simulink model "SimulinkCFARHDLWorkflowExampleNew0710"  (R2022a)
settings: Solver=FixedStepDiscrete  StartTime=0.0  StopTime=T  RelTol=1e-3
PreLoadFcn:
  | rng default;
  | 
  | %% Parameters
  | Ncell = 1000;
  | NoTrainingCells = 50; % On One Side
  | NoGuardCells = 2; %On One Side
  | ProbabilityFalseAlarm = 0.005;
  | 
  | %% Stop Time
  | tstop = Ncell;
  | Latency = NoTrainingCells + NoGuardCells + NoTrainingCells + 16 + 7;
  | T = tstop + Latency;
  | 
  | 
  | %% Input
  | x = 1/sqrt(2)*(randn(1,Ncell) + 1i*randn(1,Ncell));
  | S = [x zeros(1,Latency)]; % Padding Zeros for Streaming
  | 
  | %% Fixed Point
  | 
  | FixedPointWord = 24;
  | FractionLength = 12;
  | Signed = 1;
undefined symbols (not defined in the file): y_t1
libraries: phaseddetectlib x1
settings Model: DataTypeOverride=Off  PauseTimes=1118  Creator=The MathWorks, Inc.  LastModifiedBy=vboxuser
settings SolverCC: AlgebraicLoopSolver=TrustRegion  MaxZcPerStep=1
settings OptimizationCC: BlockReduction=off  ConditionallyExecuteInputs=off  DefaultParameterBehavior=Inlined
settings DebuggingCC: AlgebraicLoopMsg=error  SingleTaskRateTransMsg=error  IntegerOverflowMsg=none  ParameterPrecisionLossMsg=none  UnconnectedInputMsg=warning  UnconnectedOutputMsg=warning  UnconnectedLineMsg=warning  SFMachineParentedDataDiag=warning
settings HardwareCC: ProdBitPerPointer=32  ProdBitPerSizeT=32  ProdBitPerPtrDiffT=32  ProdLargestAtomicFloat=None  ProdIntDivRoundTo=Undefined  ProdEndianess=Unspecified  ProdWordSize=32  ProdHWDeviceType=ASIC/FPGA->ASIC/FPGA  TargetBitPerPointer=64  TargetBitPerSizeT=64  TargetBitPerPtrDiffT=64  TargetLongLongMode=on  TargetIntDivRoundTo=Zero  TargetEndianess=LittleEndian  TargetWordSize=64  TargetHWDeviceType=Custom Processor->MATLAB Host Computer  ProdEqTarget=off
settings RTWCC: DLArmComputeVersion=19.05

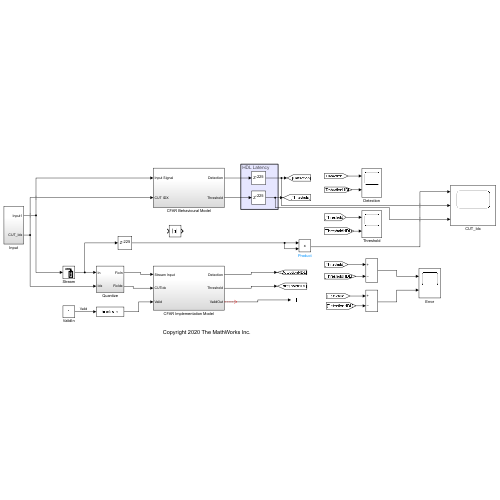
[thumbnail: Simulink's stored preview of the top-level diagram]
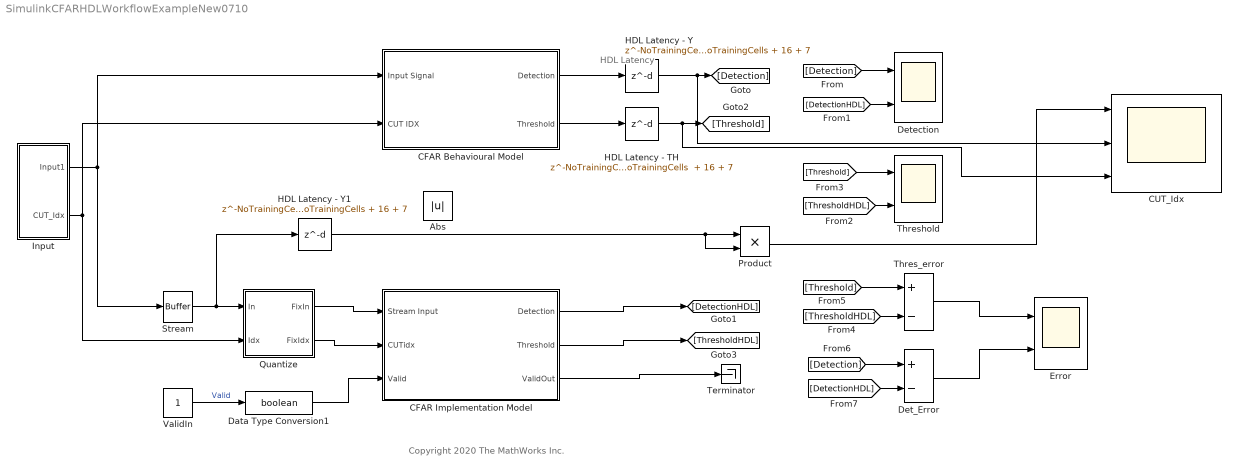
== system SimulinkCFARHDLWorkflowExampleNew0710 ==
  note: Copyright 2020 The MathWorks Inc.
  note: HDL Latency
  Abs : Abs  SaturateOnIntegerOverflow=off
  CFAR Behavioural Model : Subsystem
  CFAR Implementation Model : Subsystem
  "CUT_Idx " : Scope  NumInputPorts=3
  Data Type Conversion1 : DataTypeConversion  OutDataTypeStr=boolean  SaturateOnIntegerOverflow=off  RndMeth=Floor
  Det_Error : Sum  Inputs=+-
  Detection : Scope  NumInputPorts=2
  Error : Scope  NumInputPorts=2
  HDL Latency - TH : Delay  DelayLength="NoTrainingCells + NoGuardCells + NoTrainingCells  + 16 + 7"
  HDL Latency - Y : Delay  DelayLength=NoTrainingCells + NoGuardCells + NoTrainingCells + 16 + 7
  HDL Latency - Y1 : Delay  DelayLength=NoTrainingCells + NoGuardCells + NoTrainingCells + 16 + 7
  Input : Subsystem
  Product : Product
  Quantize : Subsystem
  Stream : Buffer  N=1  OutputFrames=off
  Terminator : Terminator
  Thres_error : Sum  Inputs=+-
  Threshold : Scope  NumInputPorts=2
  ValidIn : Constant  SampleTime=1
  wires:
  HDL Latency - Y/1 -> "CUT_Idx "/2, [Detection]
  HDL Latency - TH/1 -> "CUT_Idx "/3, [Threshold]
  Thres_error/1 -> Error/1
  Det_Error/1 -> Error/2
  [Detection] -> Detection/1
  [DetectionHDL] -> Detection/2
  [ThresholdHDL] -> Threshold/2
  [Threshold] -> Threshold/1
  [ThresholdHDL] -> Thres_error/2
  [Threshold] -> Thres_error/1
  [Detection] -> Det_Error/1
  [DetectionHDL] -> Det_Error/2
  Stream/1 -> HDL Latency - Y1/1, Quantize/1(In)
  CFAR Implementation Model/2(Threshold) -> [ThresholdHDL]
  CFAR Implementation Model/1(Detection) -> [DetectionHDL]
  Quantize/1(FixIn) -> CFAR Implementation Model/1(Stream Input)
  Quantize/2(FixIdx) -> CFAR Implementation Model/2(CUTidx)
  ValidIn/1 -> Data Type Conversion1/1  "Valid"
  CFAR Implementation Model/3(ValidOut) -> Terminator/1
  Data Type Conversion1/1 -> CFAR Implementation Model/3(Valid)
  CFAR Behavioural Model/1(Detection) -> HDL Latency - Y/1
  CFAR Behavioural Model/2(Threshold) -> HDL Latency - TH/1
  Input/1(Input1) -> CFAR Behavioural Model/1(Input Signal), Stream/1
  Input/2(CUT_Idx) -> CFAR Behavioural Model/2(CUT IDX), Quantize/2(Idx)
  Product/1 -> "CUT_Idx "/1
  HDL Latency - Y1/1 -> Product/2, Product/1
  ? -> ?

== system SimulinkCFARHDLWorkflowExampleNew0710/CFAR Behavioural Model ==
  Input Signal : Inport
  CUT IDX : Inport  Port=2
  CFAR Detector : phaseddetectlib/CFAR Detector  Method=CA  Rank=1  NumGuardCells=NoGuardCells*2  NumTrainingCells=NoTrainingCells*2  ThresholdFactor=Auto  ProbabilityFalseAlarm=ProbabilityFalseAlarm  CustomThresholdFactor=1  OutputFormat=CUT result  ThresholdOutputPort=on  NoisePowerOutputPort=off  NumDetectionsSource=Auto  NumDetections=1  SimulateUsing=Interpreted execution
      settings: SourceProductBaseCode=AR
  Selector1 : Selector  InputPortWidth=T  IndexOptions=Index vector (dialog)  Indices=1:Ncell  OutputSizes=1
  SquareLaw : Subsystem
  Detection : Outport
  Threshold : Outport  Port=2
  wires:
  CFAR Detector/1 -> Detection/1
  CFAR Detector/2 -> Threshold/1
  SquareLaw/1(SQR_LAW) -> CFAR Detector/1
  CUT IDX/1 -> CFAR Detector/2
  Input Signal/1 -> Selector1/1
  Selector1/1 -> SquareLaw/1(input)

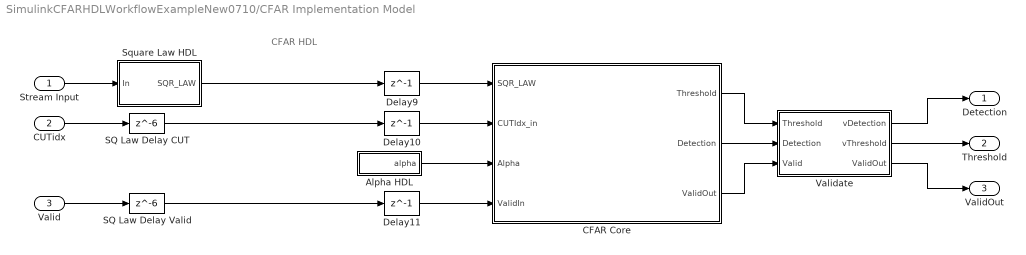
== system SimulinkCFARHDLWorkflowExampleNew0710/CFAR Implementation Model ==
  note: CFAR HDL
  Stream Input : Inport
  CUTidx : Inport  Port=2
  Valid : Inport  Port=3
  Alpha HDL : Subsystem
  CFAR Core : Subsystem
  Delay10 : Delay  DelayLength=1
  Delay11 : Delay  DelayLength=1
  Delay9 : Delay  DelayLength=1
  SQ Law Delay CUT : Delay  DelayLength=6
  SQ Law Delay Valid : Delay  DelayLength=6
  Square Law HDL : Subsystem
  Validate : Subsystem
  Detection : Outport
  Threshold : Outport  Port=2
  ValidOut : Outport  Port=3
  wires:
  Stream Input/1 -> Square Law HDL/1(In)
  Validate/3(ValidOut) -> ValidOut/1
  Validate/1(vDetection) -> Detection/1
  CUTidx/1 -> SQ Law Delay CUT/1
  Validate/2(vThreshold) -> Threshold/1
  Valid/1 -> SQ Law Delay Valid/1
  CFAR Core/3(ValidOut) -> Validate/3(Valid)
  Square Law HDL/1(SQR_LAW) -> Delay9/1
  SQ Law Delay CUT/1 -> Delay10/1
  CFAR Core/1(Threshold) -> Validate/1(Threshold)
  Alpha HDL/1(alpha) -> CFAR Core/3(Alpha)
  Delay11/1 -> CFAR Core/4(ValidIn)
  CFAR Core/2(Detection) -> Validate/2(Detection)
  Delay10/1 -> CFAR Core/2(CUTIdx_in)
  SQ Law Delay Valid/1 -> Delay11/1
  Delay9/1 -> CFAR Core/1(SQR_LAW)

== system SimulinkCFARHDLWorkflowExampleNew0710/Input ==
  CUT : Subsystem
  Input : Constant  Value=S
  Input2 : Constant  Value=y_t1
  Input1 : Outport
  CUT_Idx : Outport  Port=2
  wires:
  CUT/1(CUT_ref) -> CUT_Idx/1  "CUT_Idx"
  Input2/1 -> Input1/1  "Input"

== system SimulinkCFARHDLWorkflowExampleNew0710/Quantize ==
  In : Inport
  Idx : Inport  Port=2
  Fixed_Point_Idx : DataTypeConversion  OutDataTypeStr=fixdt(1,16,0)  SaturateOnIntegerOverflow=off  RndMeth=Floor
  Fixed_Point_Input : DataTypeConversion  OutDataTypeStr=fixdt(1,FixedPointWord,FractionLength)  SaturateOnIntegerOverflow=off  RndMeth=Floor
  FixIn : Outport
  FixIdx : Outport  Port=2
  wires:
  Fixed_Point_Input/1 -> FixIn/1
  Fixed_Point_Idx/1 -> FixIdx/1
  In/1 -> Fixed_Point_Input/1
  Idx/1 -> Fixed_Point_Idx/1

== system SimulinkCFARHDLWorkflowExampleNew0710/CFAR Behavioural Model/SquareLaw ==
  input : Inport
  Complex to Real-Imag : ComplexToRealImag
  a.a : Product
  a.a + b.b : Sum
  b.b : Product
  SQR_LAW : Outport
  wires:
  input/1 -> Complex to Real-Imag/1
  Complex to Real-Imag/2 -> b.b/1, b.b/2
  a.a/1 -> a.a + b.b/1
  a.a + b.b/1 -> SQR_LAW/1  "SQR_LAW"
  b.b/1 -> a.a + b.b/2
  Complex to Real-Imag/1 -> a.a/2, a.a/1

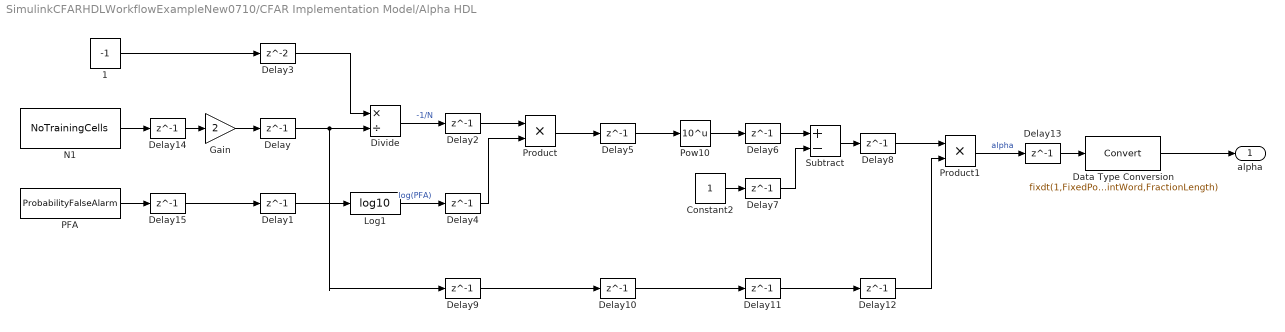
== system SimulinkCFARHDLWorkflowExampleNew0710/CFAR Implementation Model/Alpha HDL ==
  1 : Constant  Value=-1  OutDataTypeStr=Inherit: Inherit via back propagation  SampleTime=1
  Constant2 : Constant  OutDataTypeStr=Inherit: Inherit via back propagation  SampleTime=1
  Data Type Conversion : DataTypeConversion  OutDataTypeStr=fixdt(1,FixedPointWord,FractionLength)  SaturateOnIntegerOverflow=off  RndMeth=Floor
  Delay{,1..2,4..15} (15 alike) : Delay  DelayLength=1  InitialCondition=1
  Delay3 : Delay  InitialCondition=1
  Divide : Product  Inputs=*/  InputSameDT=on  RndMeth=Simplest  SaturateOnIntegerOverflow=on
  Gain : Gain  Gain=2
  Log1 : Math  Operator=log10  SignedPower=on  RndMeth=Zero
  N1 : Constant  Value=NoTrainingCells  OutDataTypeStr=single  SampleTime=1
  PFA : Constant  Value=ProbabilityFalseAlarm  OutDataTypeStr=single  SampleTime=1
  Pow10 : Math  Operator=10^u  SignedPower=on  RndMeth=Zero
  Product : Product
  Product1 : Product
  Subtract : Sum  Inputs=+-
  alpha : Outport
  wires:
  Delay13/1 -> Data Type Conversion/1
  Delay12/1 -> Product1/2
  Delay11/1 -> Delay12/1
  Delay10/1 -> Delay11/1
  Delay9/1 -> Delay10/1
  Delay8/1 -> Product1/1
  Delay7/1 -> Subtract/2
  Delay6/1 -> Subtract/1
  Delay5/1 -> Pow10/1
  Delay4/1 -> Product/2
  Delay3/1 -> Divide/1
  Delay2/1 -> Product/1
  Delay1/1 -> Log1/1
  Delay/1 -> Delay9/1, Divide/2
  N1/1 -> Delay14/1
  Product/1 -> Delay5/1
  Divide/1 -> Delay2/1  "-1/N"
  Pow10/1 -> Delay6/1
  1/1 -> Delay3/1
  Constant2/1 -> Delay7/1
  Product1/1 -> Delay13/1  "alpha"
  Log1/1 -> Delay4/1  "log(PFA)"
  Subtract/1 -> Delay8/1
  PFA/1 -> Delay15/1
  Delay14/1 -> Gain/1
  Delay15/1 -> Delay1/1
  Gain/1 -> Delay/1
  Data Type Conversion/1 -> alpha/1

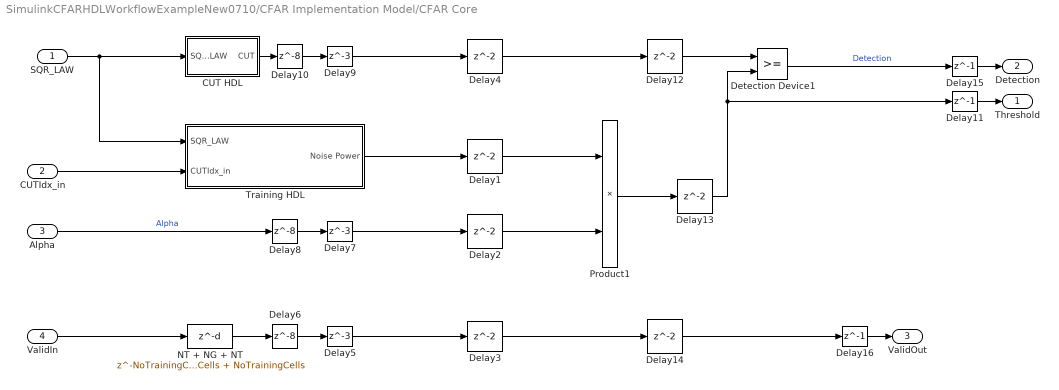
== system SimulinkCFARHDLWorkflowExampleNew0710/CFAR Implementation Model/CFAR Core ==
  SQR_LAW : Inport
  CUTIdx_in : Inport  Port=2
  Alpha : Inport  Port=3
  ValidIn : Inport  Port=4
  CUT HDL : Subsystem
  Delay{1..4,12..14} (7 alike) : Delay
  Delay10 : Delay  DelayLength=8
  Delay11 : Delay  DelayLength=1
  Delay15 : Delay  DelayLength=1
  Delay16 : Delay  DelayLength=1
  Delay5 : Delay  DelayLength=3
  Delay6 : Delay  DelayLength=8
  Delay7 : Delay  DelayLength=3
  Delay8 : Delay  DelayLength=8
  Delay9 : Delay  DelayLength=3
  Detection Device1 : RelationalOperator  OutDataTypeStr=boolean  RndMeth=Simplest
  NT + NG + NT : Delay  DelayLength=NoTrainingCells + NoGuardCells + NoTrainingCells
  Product1 : Product  InputSameDT=on  OutDataTypeStr=Inherit: Same as first input
  Training HDL : Subsystem
  Threshold : Outport
  Detection : Outport  Port=2
  ValidOut : Outport  Port=3
  wires:
  SQR_LAW/1 -> Training HDL/1(SQR_LAW), CUT HDL/1(SQR_LAW)
  Alpha/1 -> Delay8/1  "Alpha"
  Detection Device1/1 -> Delay15/1  "Detection"
  CUTIdx_in/1 -> Training HDL/2(CUTIdx_in)
  Product1/1 -> Delay13/1
  ValidIn/1 -> NT + NG + NT/1
  Delay1/1 -> Product1/1
  Delay2/1 -> Product1/2
  Delay3/1 -> Delay14/1
  Delay4/1 -> Delay12/1
  Delay6/1 -> Delay5/1
  Delay8/1 -> Delay7/1
  Delay10/1 -> Delay9/1
  NT + NG + NT/1 -> Delay6/1
  CUT HDL/1(CUT) -> Delay10/1
  Delay9/1 -> Delay4/1
  Training HDL/1(Noise Power) -> Delay1/1
  Delay7/1 -> Delay2/1
  Delay5/1 -> Delay3/1
  Delay12/1 -> Detection Device1/1
  Delay13/1 -> Delay11/1, Detection Device1/2
  Delay14/1 -> Delay16/1
  Delay15/1 -> Detection/1
  Delay11/1 -> Threshold/1
  Delay16/1 -> ValidOut/1

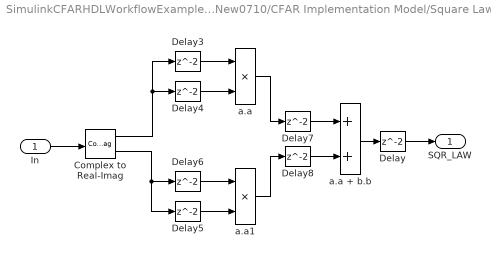
== system SimulinkCFARHDLWorkflowExampleNew0710/CFAR Implementation Model/Square Law HDL ==
  In : Inport
  Complex to Real-Imag : ComplexToRealImag
  Delay{,3..8} (7 alike) : Delay
  a.a : Product  InputSameDT=on  OutDataTypeStr=fixdt(1,FixedPointWord,FractionLength)
  a.a + b.b : Sum  InputSameDT=on  OutDataTypeStr=fixdt(1,FixedPointWord,FractionLength)
  a.a1 : Product  InputSameDT=on  OutDataTypeStr=fixdt(1,FixedPointWord,FractionLength)
  SQR_LAW : Outport
  wires:
  Delay7/1 -> a.a + b.b/1
  a.a + b.b/1 -> Delay/1
  Delay5/1 -> a.a1/2
  Complex to Real-Imag/2 -> Delay6/1, Delay5/1
  Complex to Real-Imag/1 -> Delay4/1, Delay3/1
  Delay8/1 -> a.a + b.b/2
  Delay3/1 -> a.a/1
  a.a/1 -> Delay7/1
  a.a1/1 -> Delay8/1
  Delay4/1 -> a.a/2
  Delay6/1 -> a.a1/1
  Delay/1 -> SQR_LAW/1
  In/1 -> Complex to Real-Imag/1

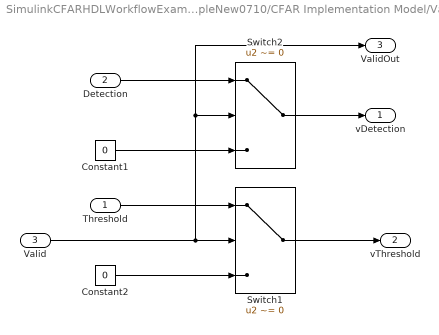
== system SimulinkCFARHDLWorkflowExampleNew0710/CFAR Implementation Model/Validate ==
  Threshold : Inport
  Detection : Inport  Port=2
  Valid : Inport  Port=3
  Constant1 : Constant  Value=0  OutDataTypeStr=boolean  SampleTime=1
  Constant2 : Constant  Value=0  OutDataTypeStr=Inherit: Inherit via back propagation  SampleTime=1
  Switch1 : Switch  Criteria=u2 ~= 0  Threshold=1  OutDataTypeStr=fixdt(1,12,8)  SaturateOnIntegerOverflow=off
  Switch2 : Switch  Criteria=u2 ~= 0  Threshold=1  OutDataTypeStr=boolean  SaturateOnIntegerOverflow=off
  vDetection : Outport
  vThreshold : Outport  Port=2
  ValidOut : Outport  Port=3
  wires:
  Valid/1 -> ValidOut/1, Switch2/2, Switch1/2
  Switch1/1 -> vThreshold/1
  Constant2/1 -> Switch1/3
  Threshold/1 -> Switch1/1
  Switch2/1 -> vDetection/1
  Detection/1 -> Switch2/1
  Constant1/1 -> Switch2/3

== system SimulinkCFARHDLWorkflowExampleNew0710/Input/CUT ==
  Data Type Conversion1 : DataTypeConversion  OutDataTypeStr=double  SaturateOnIntegerOverflow=off  RndMeth=Floor  LockScale=on
  UpCounter : Subsystem
  CUT_ref : Outport
  wires:
  Data Type Conversion1/1 -> CUT_ref/1  "CUT_ref"
  UpCounter/1(Count) -> Data Type Conversion1/1

== system SimulinkCFARHDLWorkflowExampleNew0710/CFAR Implementation Model/CFAR Core/CUT HDL ==
  SQR_LAW : Inport
  Delay2 : Delay  DelayLength=NoTrainingCells + NoGuardCells + NoTrainingCells
  CUT : Outport
  wires:
  Delay2/1 -> CUT/1  "CUT"
  SQR_LAW/1 -> Delay2/1

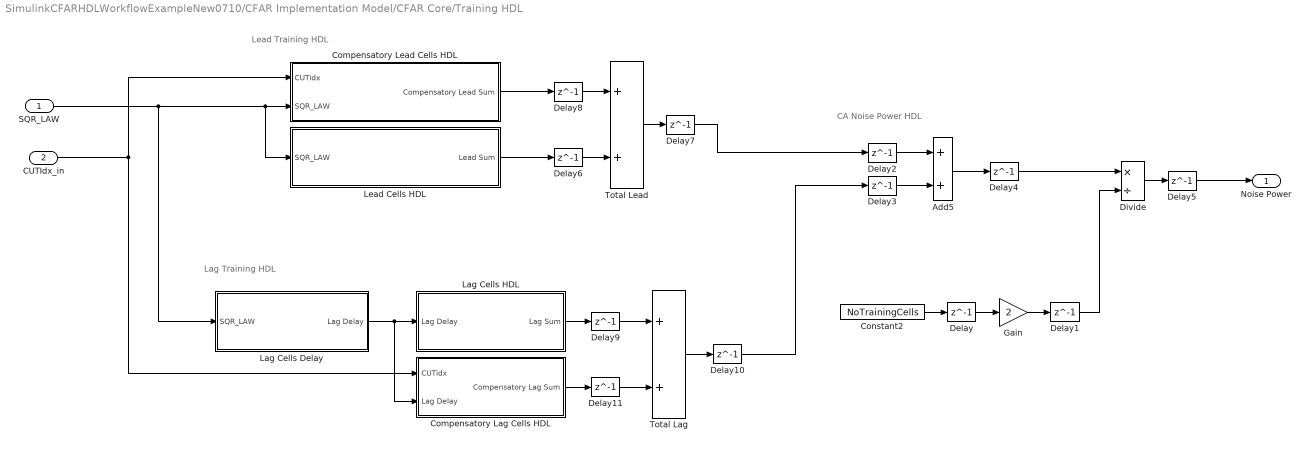
== system SimulinkCFARHDLWorkflowExampleNew0710/CFAR Implementation Model/CFAR Core/Training HDL ==
  note: Lag Training HDL
  note: Lead Training HDL
  note: CA Noise Power HDL
  SQR_LAW : Inport
  CUTIdx_in : Inport  Port=2
  Add5 : Sum  InputSameDT=on  OutDataTypeStr=Inherit: Same as accumulator  SaturateOnIntegerOverflow=on
  Compensatory Lag Cells HDL : Subsystem
  Compensatory Lead Cells HDL : Subsystem
  Constant2 : Constant  Value=NoTrainingCells  OutDataTypeStr=int16  SampleTime=1
  Delay : Delay  DelayLength=1  InitialCondition=1
  Delay1 : Delay  DelayLength=1  InitialCondition=1
  Delay{2..11} (10 alike) : Delay  DelayLength=1  InitialCondition=0
  Divide : Product  Inputs=*/  OutDataTypeStr=fixdt(1,FixedPointWord,FractionLength)  RndMeth=Simplest  SaturateOnIntegerOverflow=on
  Gain : Gain  Gain=2  OutDataTypeStr=int16
  Lag Cells Delay : Subsystem
  Lag Cells HDL : Subsystem
  Lead Cells HDL : Subsystem
  Total Lag : Sum  InputSameDT=on  AccumDataTypeStr=fixdt(1,FixedPointWord,FractionLength)  OutDataTypeStr=Inherit: Same as accumulator  SaturateOnIntegerOverflow=on
  Total Lead : Sum  InputSameDT=on  AccumDataTypeStr=fixdt(1,FixedPointWord,FractionLength)  OutDataTypeStr=Inherit: Same as accumulator  SaturateOnIntegerOverflow=on
  Noise Power : Outport
  wires:
  Delay5/1 -> Noise Power/1
  Delay4/1 -> Divide/1
  Delay3/1 -> Add5/2
  Delay2/1 -> Add5/1
  Delay1/1 -> Divide/2
  Delay/1 -> Gain/1
  Add5/1 -> Delay4/1
  Divide/1 -> Delay5/1
  Delay10/1 -> Delay3/1
  Gain/1 -> Delay1/1
  Constant2/1 -> Delay/1
  Delay7/1 -> Delay2/1
  Delay6/1 -> Total Lead/2
  Delay8/1 -> Total Lead/1
  Total Lead/1 -> Delay7/1
  Compensatory Lead Cells HDL/1(Compensatory Lead Sum) -> Delay8/1
  Lead Cells HDL/1(Lead Sum) -> Delay6/1
  Delay9/1 -> Total Lag/1
  Delay11/1 -> Total Lag/2
  SQR_LAW/1 -> Lead Cells HDL/1(SQR_LAW), Compensatory Lead Cells HDL/2(SQR_LAW), Lag Cells Delay/1(SQR_LAW)
  Total Lag/1 -> Delay10/1
  Lag Cells HDL/1(Lag Sum) -> Delay9/1
  CUTIdx_in/1 -> Compensatory Lead Cells HDL/1(CUTidx), Compensatory Lag Cells HDL/1(CUTidx)
  Lag Cells Delay/1(Lag Delay) -> Lag Cells HDL/1(Lag Delay), Compensatory Lag Cells HDL/2(Lag Delay)
  Compensatory Lag Cells HDL/1(Compensatory Lag Sum) -> Delay11/1

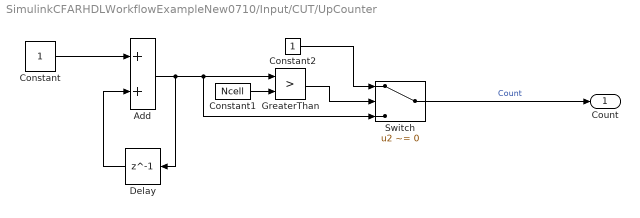
== system SimulinkCFARHDLWorkflowExampleNew0710/Input/CUT/UpCounter ==
  Add : Sum
  Constant : Constant
  Constant1 : Constant  Value=Ncell
  Constant2 : Constant
  Delay : Delay  DelayLength=1
  GreaterThan : RelationalOperator  Operator=>  OutDataTypeStr=boolean  RndMeth=Simplest  InputSameDT=off
  Switch : Switch  Criteria=u2 ~= 0  SaturateOnIntegerOverflow=off  InputSameDT=off
  Count : Outport
  wires:
  Delay/1 -> Add/2
  Add/1 -> Switch/3, GreaterThan/1, Delay/1
  Constant2/1 -> Switch/1
  Constant1/1 -> GreaterThan/2
  Constant/1 -> Add/1
  GreaterThan/1 -> Switch/2
  Switch/1 -> Count/1  "Count"

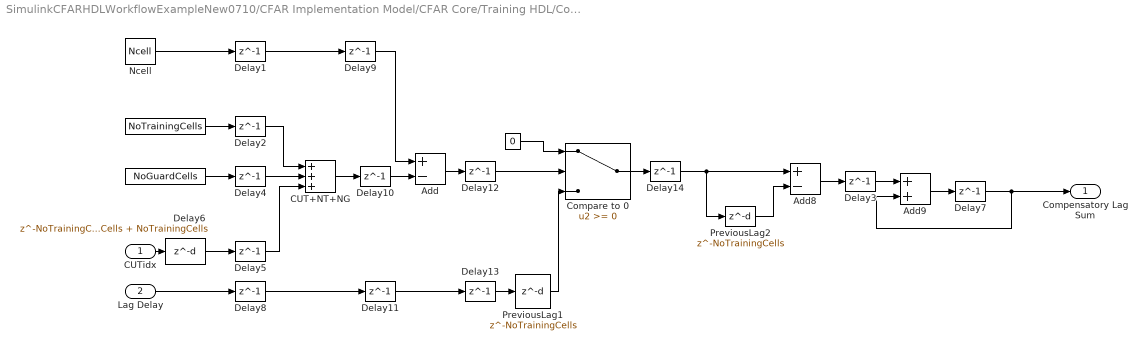
== system SimulinkCFARHDLWorkflowExampleNew0710/CFAR Implementation Model/CFAR Core/Training HDL/Compensatory Lag Cells HDL ==
  CUTidx : Inport
  Lag Delay : Inport  Port=2
  "  " : Constant  Value=0  OutDataTypeStr=fixdt(1,FixedPointWord,FractionLength)  SampleTime=1
  "    " : Constant  Value=NoGuardCells  OutDataTypeStr=int16  SampleTime=1
  "      " : Constant  Value=NoTrainingCells  OutDataTypeStr=int16  SampleTime=1
  Add : Sum  Inputs=+-  InputSameDT=on  AccumDataTypeStr=int16  OutDataTypeStr=Inherit: Same as accumulator
  Add8 : Sum  Inputs=+-  InputSameDT=on  AccumDataTypeStr=fixdt(1,FixedPointWord,FractionLength)  OutDataTypeStr=Inherit: Same as accumulator
  Add9 : Sum  InputSameDT=on  AccumDataTypeStr=fixdt(1,FixedPointWord,FractionLength)  OutDataTypeStr=Inherit: Same as accumulator  SaturateOnIntegerOverflow=on
  CUT+NT+NG : Sum  Inputs=+++  InputSameDT=on  AccumDataTypeStr=int16  OutDataTypeStr=int16
  Compare to 0 : Switch  OutDataTypeStr=fixdt(1,FixedPointWord,FractionLength)  SaturateOnIntegerOverflow=off
  Delay{1..5,7..14} (13 alike) : Delay  DelayLength=1  InitialCondition=0
  Delay6 : Delay  DelayLength=NoTrainingCells + NoGuardCells + NoTrainingCells
  Ncell : Constant  Value=Ncell  OutDataTypeStr=int16  SampleTime=1
  PreviousLag1 : Delay  DelayLength=NoTrainingCells
  PreviousLag2 : Delay  DelayLength=NoTrainingCells
  Compensatory Lag Sum : Outport
  wires:
  "    "/1 -> Delay4/1
  CUT+NT+NG/1 -> Delay10/1
  "      "/1 -> Delay2/1
  PreviousLag1/1 -> Compare to 0/3
  Delay6/1 -> Delay5/1
  Lag Delay/1 -> Delay8/1
  Add8/1 -> Delay3/1
  "  "/1 -> Compare to 0/1
  Ncell/1 -> Delay1/1
  CUTidx/1 -> Delay6/1
  Compare to 0/1 -> Delay14/1
  PreviousLag2/1 -> Add8/2
  Delay3/1 -> Add9/1
  Add9/1 -> Delay7/1
  Delay7/1 -> Compensatory Lag Sum/1, Add9/2
  Delay1/1 -> Delay9/1
  Delay2/1 -> CUT+NT+NG/1
  Delay4/1 -> CUT+NT+NG/2
  Delay5/1 -> CUT+NT+NG/3
  Delay8/1 -> Delay11/1
  Delay9/1 -> Add/1
  Delay10/1 -> Add/2
  Delay11/1 -> Delay13/1
  Add/1 -> Delay12/1
  Delay12/1 -> Compare to 0/2
  Delay13/1 -> PreviousLag1/1
  Delay14/1 -> Add8/1, PreviousLag2/1

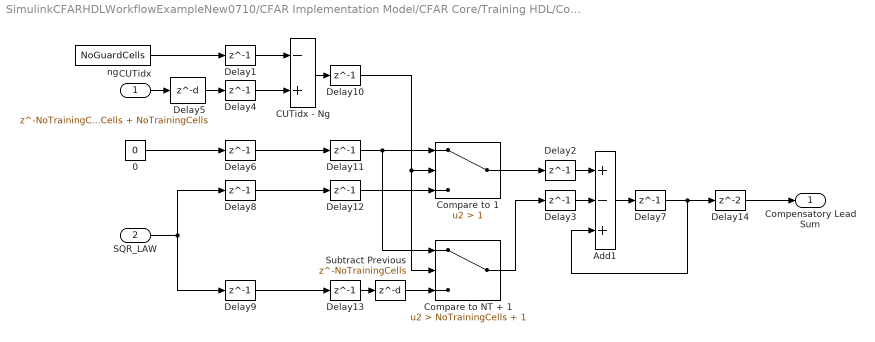
== system SimulinkCFARHDLWorkflowExampleNew0710/CFAR Implementation Model/CFAR Core/Training HDL/Compensatory Lead Cells HDL ==
  CUTidx : Inport
  SQR_LAW : Inport  Port=2
  0 : Constant  Value=0  OutDataTypeStr=Inherit: Inherit via back propagation  SampleTime=1
  Add1 : Sum  Inputs=+-+  InputSameDT=on  AccumDataTypeStr=fixdt(1,FixedPointWord,FractionLength)  OutDataTypeStr=Inherit: Same as accumulator  SaturateOnIntegerOverflow=on
  CUTidx - Ng : Sum  Inputs=-+  InputSameDT=on  AccumDataTypeStr=int16  OutDataTypeStr=int16
  Compare to 1 : Switch  Criteria=u2 > Threshold  Threshold=1  SaturateOnIntegerOverflow=off  InputSameDT=off
  Compare to NT + 1 : Switch  Criteria=u2 > Threshold  Threshold=NoTrainingCells + 1  ZeroCross=off  SaturateOnIntegerOverflow=off  InputSameDT=off
  Delay{1..4,6..13} (12 alike) : Delay  DelayLength=1  InitialCondition=0
  Delay14 : Delay  InitialCondition=0
  Delay5 : Delay  DelayLength=NoTrainingCells + NoGuardCells + NoTrainingCells
  Subtract Previous : Delay  DelayLength=NoTrainingCells
  ng : Constant  Value=NoGuardCells  OutDataTypeStr=Inherit: Inherit via back propagation  SampleTime=1
  Compensatory Lead Sum : Outport
  wires:
  Compare to 1/1 -> Delay2/1
  CUTidx - Ng/1 -> Delay10/1
  SQR_LAW/1 -> Delay9/1, Delay8/1
  Subtract Previous/1 -> Compare to NT + 1/3
  ng/1 -> Delay1/1
  Delay7/1 -> Add1/3, Delay14/1
  Delay5/1 -> Delay4/1
  0/1 -> Delay6/1
  Compare to NT + 1/1 -> Delay3/1
  CUTidx/1 -> Delay5/1
  Delay2/1 -> Add1/1
  Delay3/1 -> Add1/2
  Add1/1 -> Delay7/1
  Delay1/1 -> CUTidx - Ng/1
  Delay4/1 -> CUTidx - Ng/2
  Delay6/1 -> Delay11/1
  Delay8/1 -> Delay12/1
  Delay9/1 -> Delay13/1
  Delay10/1 -> Compare to NT + 1/2, Compare to 1/2
  Delay11/1 -> Compare to NT + 1/1, Compare to 1/1
  Delay12/1 -> Compare to 1/3
  Delay13/1 -> Subtract Previous/1
  Delay14/1 -> Compensatory Lead Sum/1

== system SimulinkCFARHDLWorkflowExampleNew0710/CFAR Implementation Model/CFAR Core/Training HDL/Lag Cells Delay ==
  SQR_LAW : Inport
  CUT : Delay  DelayLength=1
  GuardLag : Delay  DelayLength=NoGuardCells
  GuardLead : Delay  DelayLength=NoGuardCells
  PreTraining Comp : Delay  DelayLength=NoTrainingCells
  Training : Delay  DelayLength=NoTrainingCells
  Lag Delay : Outport
  wires:
  Training/1 -> GuardLag/1
  PreTraining Comp/1 -> Training/1
  SQR_LAW/1 -> PreTraining Comp/1
  CUT/1 -> GuardLead/1
  GuardLag/1 -> CUT/1
  GuardLead/1 -> Lag Delay/1  "Lag Delay"

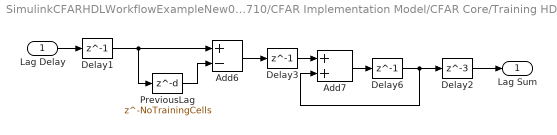
== system SimulinkCFARHDLWorkflowExampleNew0710/CFAR Implementation Model/CFAR Core/Training HDL/Lag Cells HDL ==
  Lag Delay : Inport
  Add6 : Sum  Inputs=+-  InputSameDT=on  AccumDataTypeStr=fixdt(1,FixedPointWord,FractionLength)  OutDataTypeStr=Inherit: Same as accumulator
  Add7 : Sum  InputSameDT=on  AccumDataTypeStr=fixdt(1,FixedPointWord,FractionLength)  SaturateOnIntegerOverflow=on  OutDataTypeStr=Inherit: Same as first input
  Delay1 : Delay  DelayLength=1  InitialCondition=0
  Delay2 : Delay  DelayLength=3  InitialCondition=0
  Delay3 : Delay  DelayLength=1  InitialCondition=0
  Delay6 : Delay  DelayLength=1  InitialCondition=0
  PreviousLag : Delay  DelayLength=NoTrainingCells
  Lag Sum : Outport
  wires:
  Add6/1 -> Delay3/1
  Lag Delay/1 -> Delay1/1
  PreviousLag/1 -> Add6/2
  Delay3/1 -> Add7/1
  Add7/1 -> Delay6/1
  Delay6/1 -> Add7/2, Delay2/1
  Delay1/1 -> Add6/1, PreviousLag/1
  Delay2/1 -> Lag Sum/1

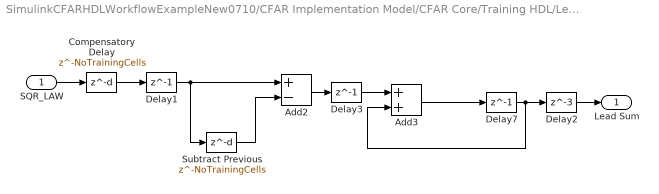
== system SimulinkCFARHDLWorkflowExampleNew0710/CFAR Implementation Model/CFAR Core/Training HDL/Lead Cells HDL ==
  SQR_LAW : Inport
  Add2 : Sum  Inputs=+-  AccumDataTypeStr=fixdt(1,FixedPointWord,FractionLength)  OutDataTypeStr=Inherit: Same as accumulator
  Add3 : Sum  AccumDataTypeStr=fixdt(1,FixedPointWord,FractionLength)  OutDataTypeStr=Inherit: Same as accumulator  SaturateOnIntegerOverflow=on
  Compensatory Delay : Delay  DelayLength=NoTrainingCells
  Delay1 : Delay  DelayLength=1  InitialCondition=0
  Delay2 : Delay  DelayLength=3  InitialCondition=0
  Delay3 : Delay  DelayLength=1  InitialCondition=0
  Delay7 : Delay  DelayLength=1  InitialCondition=0
  Subtract Previous : Delay  DelayLength=NoTrainingCells
  Lead Sum : Outport
  wires:
  SQR_LAW/1 -> Compensatory Delay/1
  Add2/1 -> Delay3/1
  Compensatory Delay/1 -> Delay1/1
  Subtract Previous/1 -> Add2/2
  Delay3/1 -> Add3/1
  Add3/1 -> Delay7/1
  Delay7/1 -> Delay2/1, Add3/2
  Delay1/1 -> Add2/1, Subtract Previous/1
  Delay2/1 -> Lead Sum/1
